simulink model "Battery_Model"  (R2025b)
settings: Solver=VariableStepAuto  StartTime=0.0  StopTime=3000  MaxStep=0.1  MinStep=0.0001  RelTol=1e-3
undefined symbols (not defined in the file or in its folder): DiscIntNeverNeededParam
settings Model: Creator=gonza  LastModifiedBy=gonza

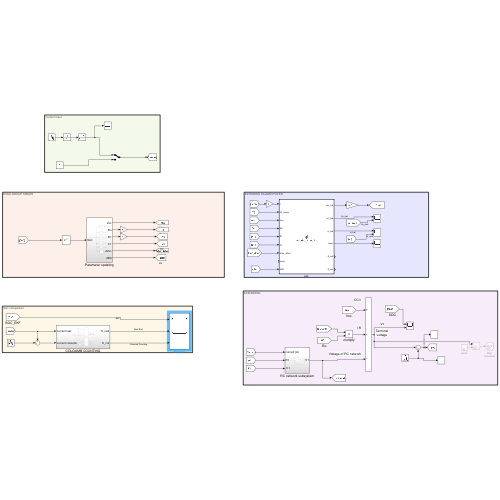
[thumbnail: Simulink's stored preview of the top-level diagram]
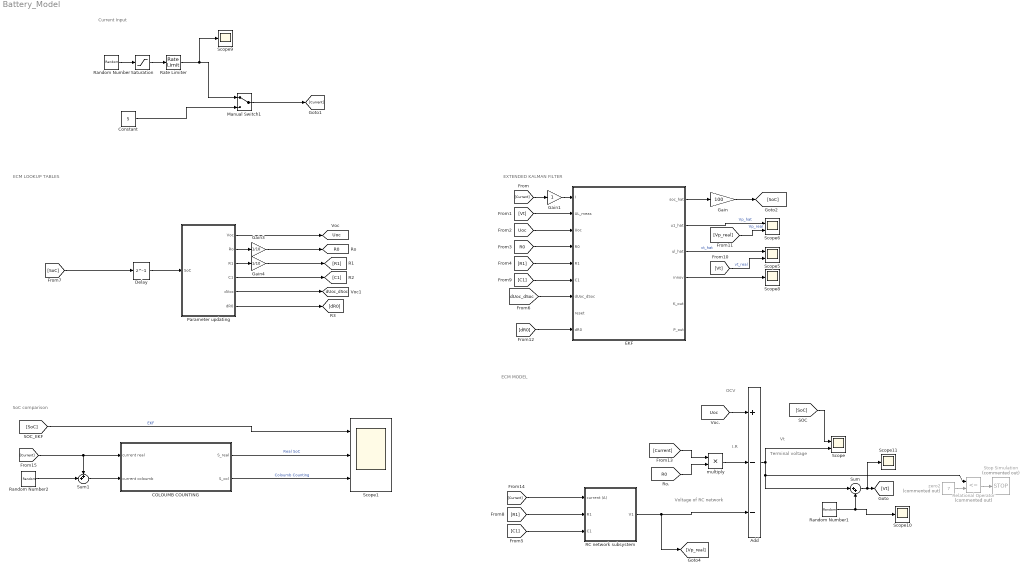
== system Battery_Model ==
  note: SoC comparison
  note: ECM MODEL
  note: Current Input
  note: ECM LOOKUP TABLES
  note: EXTENDED KALMAN FILTER
  note: OCV
  note: Terminal
      |  voltage
  note: Voltage of RC network
  note: Vt
  note: I.R
  Add : Sum  Inputs=+--
  COLOUMB COUNTING : Subsystem
  Constant : Constant  Value=5
  Delay : Delay  DelayLength=1  InitialCondition=80  InputProcessing=Columns as channels (frame based)
  EKF : MATLAB Function  TreatAsAtomicUnit=on
  Gain : Gain  Gain=100
  Gain1 : Gain
  Gain3 : Gain  Gain=1/10
  Gain4 : Gain  Gain=1/10
  Manual Switch1 : ManualSwitch
  Parameter updating : Subsystem
  RC network subsystem : Subsystem
  Random Number : RandomNumber  Variance=100  SampleTime=5
  Random Number1 : RandomNumber  Variance=0.00001  Seed=10  SampleTime=0.01
  Random Number2 : RandomNumber  Variance=0.01  Seed=123412  SampleTime=0.01
  Rate Limiter : RateLimiter  RisingSlewLimit=100  FallingSlewLimit=-100
  Relational Operator : RelationalOperator  Commented=on  Operator=<=  OutDataTypeStr=boolean  InputSameDT=off
  Saturation : Saturate  UpperLimit=100  LowerLimit=-1
  Scope : Scope  NumInputPorts=2
      settings: ActiveDisplayYMinimum=-7.8038423076394752  ActiveDisplayYMaximum=89.71598082300477
  Scope1 : Scope  NumInputPorts=3
      settings: ActiveDisplayYMinimum=5.9960554077224213  ActiveDisplayYMaximum=88.222660510253064
  Scope{8..11} (4 alike) : Scope
      Scope10 settings: ActiveDisplayYMinimum=-0.017996200767772353  ActiveDisplayYMaximum=0.017647380035145821  DataLoggingVariableName=ScopeData10
      Scope11 settings: ActiveDisplayYMinimum=7.0317837281458875  ActiveDisplayYMaximum=7.8836427087263461  DataLoggingVariableName=ScopeData11
      Scope8 settings: ActiveDisplayYMinimum=-0.017332160959111498  ActiveDisplayYMaximum=0.016983840592250665  DataLoggingVariableName=ScopeData8
      Scope9 settings: ActiveDisplayYMinimum=-7.4624542671868479  ActiveDisplayYMaximum=23.142723507063309  DataLoggingVariableName=ScopeData9
  Scope5 : Scope  NumInputPorts=2
      settings: ActiveDisplayYMinimum=7.1842164891272571  ActiveDisplayYMaximum=7.98783766896863  DataLoggingVariableName=ScopeData5
  Scope6 : Scope  NumInputPorts=2
      settings: ActiveDisplayYMinimum=-0.0084839213010874728  ActiveDisplayYMaximum=0.076355291709787276  DataLoggingVariableName=ScopeData6
  Stop Simulation : Stop  Commented=on
  Sum : Sum  Inputs=|++
  Sum1 : Sum  Inputs=++|
  multiply : Product  Inputs=**
  zero2 : Constant  Commented=on  Value=7
  tag scope: R0=global, Uoc=global, dUoc_dSoc=global
  wires:
  EKF/4(innov) -> Scope8/1
  Gain1/1 -> EKF/1(I)
  [dUoc_dSoc] -> EKF/7(dUoc_dSoc)
  EKF/1(soc_hat) -> Gain/1
  Gain/1 -> [SoC]
  [Current] -> Gain1/1
  [R0] -> EKF/4(R0)
  [Vt] -> EKF/2(UL_meas)
  [dR0] -> EKF/9(dR0)
  [C1] -> EKF/6(C1)
  [R1] -> EKF/5(R1)
  EKF/2(u1_hat) -> Scope6/1  "Vp_hat"
  EKF/3(ul_hat) -> Scope5/1  "vt_hat"
  [Vt] -> Scope5/2  "vt_real"
  [Vp_real] -> Scope6/2  "Vp_real"
  [Uoc] -> EKF/3(Uoc)
  Parameter updating/2(Ro) -> Gain3/1
  Gain3/1 -> [R0]
  Parameter updating/1(Voc) -> [Uoc]
  Parameter updating/3(R1) -> Gain4/1
  Gain4/1 -> [R1]
  Parameter updating/5(dVoc) -> [dUoc_dSoc]
  Parameter updating/6(dR0) -> [dR0]
  [SoC] -> Delay/1
  Parameter updating/4(C1) -> [C1]
  Delay/1 -> Parameter updating/1(SoC)
  Constant/1 -> Manual Switch1/2
  Random Number/1 -> Saturation/1
  Saturation/1 -> Rate Limiter/1
  Manual Switch1/1 -> [Current]
  Rate Limiter/1 -> Scope9/1, Manual Switch1/1
  [Current] -> RC network subsystem/1(current (A))
  zero2/1 -> Relational Operator/2
  [R0] -> multiply/2
  [Uoc] -> Add/1
  Random Number1/1 -> Sum/2, Scope10/1
  Add/1 -> Relational Operator/1, Sum/1, Scope/2
  [SoC] -> Scope/1
  multiply/1 -> Add/2
  Sum/1 -> Scope11/1, [Vt]
  Relational Operator/1 -> Stop Simulation/1
  [Current] -> multiply/1
  [R1] -> RC network subsystem/2(R1)
  [C1] -> RC network subsystem/3(" C1")
  RC network subsystem/1(V1) -> Add/3, [Vp_real]
  Sum1/1 -> COLOUMB COUNTING/2(current coloumb)
  Random Number2/1 -> Sum1/2
  [SoC] -> Scope1/1  "EKF"
  [Current] -> Sum1/1, COLOUMB COUNTING/1(current real)
  COLOUMB COUNTING/1(S_real) -> Scope1/2  "Real SoC"
  COLOUMB COUNTING/2(S_col) -> Scope1/3  "Coloumb Counting"

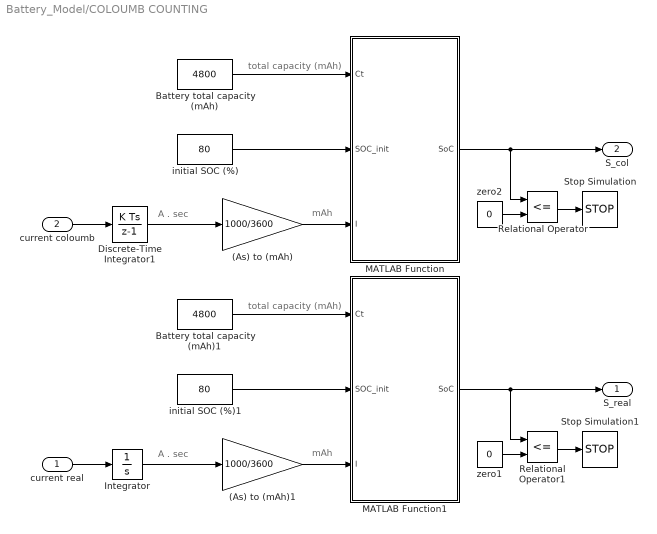
== system Battery_Model/COLOUMB COUNTING ==
  note: total capacity (mAh)
  note: A . sec
  note: mAh
  note: A . sec
  note: total capacity (mAh)
  note: mAh
  current real : Inport
  current coloumb : Inport  Port=2
  (As) to (mAh) : Gain  Gain=1000/3600
  (As) to (mAh)1 : Gain  Gain=1000/3600
  Battery total capacity (mAh) : Constant  Value=4800
  Battery total capacity (mAh)1 : Constant  Value=4800
  Discrete-Time Integrator1 : DiscreteIntegrator  ICPrevOutput=DiscIntNeverNeededParam  ICPrevScaledInput=DiscIntNeverNeededParam
  Integrator : Integrator
  MATLAB Function : MATLAB Function  TreatAsAtomicUnit=on
  MATLAB Function1 : MATLAB Function  TreatAsAtomicUnit=on
  Relational Operator : RelationalOperator  Operator=<=  OutDataTypeStr=boolean  InputSameDT=off
  Relational Operator1 : RelationalOperator  Operator=<=  OutDataTypeStr=boolean  InputSameDT=off
  Stop Simulation : Stop
  Stop Simulation1 : Stop
  initial SOC (%) : Constant  Value=80
  initial SOC (%)1 : Constant  Value=80
  zero1 : Constant  Value=0
  zero2 : Constant  Value=0
  S_real : Outport
  S_col : Outport  Port=2
  wires:
  MATLAB Function/1(SoC) -> S_col/1, Relational Operator/1
  (As) to (mAh)/1 -> MATLAB Function/3(I)
  current coloumb/1 -> Discrete-Time Integrator1/1
  Relational Operator/1 -> Stop Simulation/1
  Battery total capacity (mAh)/1 -> MATLAB Function/1(Ct)
  initial SOC (%)/1 -> MATLAB Function/2(SOC_init)
  zero2/1 -> Relational Operator/2
  zero1/1 -> Relational Operator1/2
  Relational Operator1/1 -> Stop Simulation1/1
  initial SOC (%)1/1 -> MATLAB Function1/2(SOC_init)
  current real/1 -> Integrator/1
  Battery total capacity (mAh)1/1 -> MATLAB Function1/1(Ct)
  (As) to (mAh)1/1 -> MATLAB Function1/3(I)
  MATLAB Function1/1(SoC) -> S_real/1, Relational Operator1/1
  Integrator/1 -> (As) to (mAh)1/1
  Discrete-Time Integrator1/1 -> (As) to (mAh)/1

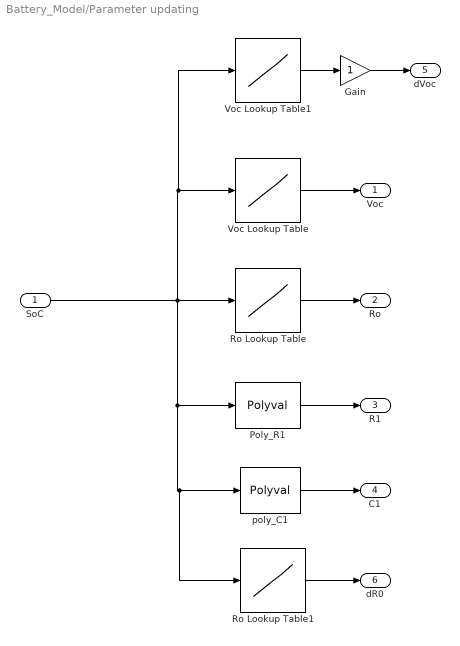
== system Battery_Model/Parameter updating ==
  SoC : Inport
  Gain : Gain
  Poly_R1 : Polyval  Coefs=[1.466124009149211e-08,-3.016114306306107e-06,2.169854530489312e-04,-0.006504304448579,0.091010234125850]
  Ro Lookup Table : Lookup_n-D  NumberOfTableDimensions=1  BreakpointsForDimension1="[0\t5\t7\t9\t11\t13\t15\t17\t19\t21\t23\t25\t27\t29\t31\t33\t35\t37\t39\t41\t43\t45\t47\t49\t51\t53\t55\t57\t59\t61\t63\t65\t67\t69\t71\t73\t75\t77\t79\t81\t83\t85\t87\t89\t91\t93\t95\t97\t100]"  Table="[0.140000000000000\t0.110000000000000\t0.110000000000000\t0.100000000000000\t0.0900000000000000\t0.0900000000000000\t0.0800000000000000\t0.0800000000000000\t0.0700000000000000\t0.0700000000000000\t0.0700000000000000\t0.0700000000000000\t0.0700000000000000\t0.0700000000000000\t0.0700000000000000\t0.0700000000000000\t0.0700000000000000\t0.0600000000000000\t0.0700000000000000\t0.0600000000000000\t0.0600000000000000\t0.0700000000000000\t0.0600000000000000\t0.0700000000000000\t0.0610000000000000\t0.0620000000000000\t0.0630000000000000\t0.0640000000000000\t0.0660000000000000\t0.0650000000000000\t0.0670000000000000\t0.0610000000000000\t0.0610000000000000\t0.0620000000000000\t0.0630000000000000\t0.0620000000000000\t0.0640000000000000\t0.0640000000000000\t0.0650000000000000\t0.0640000000000000\t0.0680000000000000\t0.0710000000000000\t0.0710000000000000\t0.0720000000000000\t0.0740000000000000\t0.0740000000000000\t0.0740000000000000\t0.0750000000000000\t0.0770000000000000]"  InternalRulePriority=Speed  RndMeth=Simplest
  Ro Lookup Table1 : Lookup_n-D  NumberOfTableDimensions=1  BreakpointsForDimension1=[0 5 7 9 11 13 15 17 19 21 23 25 27 29 31 33 35 37 39 41 43 45 47 49 51 53 55 57 59 61 63 65 67 69 71 73 75 77 79 81 83 85 87 89 91 93 95 97 100]  Table=[-0.59999999999999998 -0.42857142857142899 -0.25 -0.5 -0.25 -0.25 -0.25 -0.25 -0.25 0 0 0 0 0 0 0 -0.25 0 0 -0.25 0.25 0 0 0.025000000000000001 -0.20000000000000001 0.050000000000000003 0.050000000000000003 0.074999999999999997 0.025000000000000001 0.025000000000000001 -0.10000000000000001 -0.14999999999999999 0.025000000000000001 0.050000000000000003 0 0.025000000000000001 0.050000000000000003 0.025000000000000001 0 0.074999999999999997 0.17499999999999999 0.074999999999999997 0.025000000000000001 0.074999999999999997 0.050000000000000003 0 0.025000000000000001 0.059999999999999998 0.066666666666666999]  InternalRulePriority=Speed  RndMeth=Simplest
  Voc Lookup Table : Lookup_n-D  NumberOfTableDimensions=1  BreakpointsForDimension1="[0\t5\t7\t9\t11\t13\t15\t17\t19\t21\t23\t25\t27\t29\t31\t33\t35\t37\t39\t41\t43\t45\t47\t49\t51\t53\t55\t57\t59\t61\t63\t65\t67\t69\t71\t73\t75\t77\t79\t81\t83\t85\t87\t89\t91\t93\t95\t97\t100]"  Table="[7.01000000000000\t7.09000000000000\t7.16000000000000\t7.20000000000000\t7.29000000000000\t7.34000000000000\t7.38000000000000\t7.41000000000000\t7.44000000000000\t7.47000000000000\t7.49000000000000\t7.52000000000000\t7.54000000000000\t7.56000000000000\t7.58000000000000\t7.60000000000000\t7.61000000000000\t7.63000000000000\t7.64000000000000\t7.65000000000000\t7.66000000000000\t7.67000000000000\t7.68000000000000\t7.69000000000000\t7.69800000000000\t7.70200000000000\t7.71100000000000\t7.71400000000000\t7.72000000000000\t7.72800000000000\t7.73500000000000\t7.74000000000000\t7.74500000000000\t7.75400000000000\t7.75800000000000\t7.76100000000000\t7.76800000000000\t7.77500000000000\t7.77800000000000\t7.79000000000000\t7.80900000000000\t7.85100000000000\t7.87000000000000\t7.92300000000000\t7.98100000000000\t8.05500000000000\t8.15200000000000\t8.26600000000000\t8.44300000000000]"  InternalRulePriority=Speed  RndMeth=Simplest
  Voc Lookup Table1 : Lookup_n-D  NumberOfTableDimensions=1  BreakpointsForDimension1=[0 5 7 9 11 13 15 17 19 21 23 25 27 29 31 33 35 37 39 41 43 45 47 49 51 53 55 57 59 61 63 65 67 69 71 73 75 77 79 81 83 85 87 89 91 93 95 97 100]  Table=[1.600000000000001 2.142857142857148 2.750000000000008 3.249999999999998 3.499999999999991 2.249999999999997 1.750000000000007 1.500000000000012 1.499999999999991 1.249999999999995 1.249999999999995 1.249999999999995 1.000000000000001 1.000000000000001 1 0.750000000000007 0.750000000000007 0.749999999999983 0.500000000000012 0.500000000000012 0.499999999999989 0.49999999999999 0.500000000000012 0.450000000000017 0.299999999999989 0.324999999999997 0.300000000000012 0.224999999999987 0.349999999999983 0.375000000000014 0.300000000000011 0.249999999999994 0.349999999999984 0.324999999999998 0.175000000000014 0.249999999999994 0.350000000000006 0.249999999999994 0.374999999999992 0.775000000000016 1.525000000000001 1.524999999999997 1.8 2.774999999999991 3.299999999999989 4.274999999999992 5.275000000000017 5.820000000000002 5.899999999999982]  InternalRulePriority=Speed  RndMeth=Simplest
  poly_C1 : Polyval  Coefs=[-6.954272499766545e-05,0.013572818088594,-0.971124742038101,33.500516588178876,92.374565325126170]
  Voc : Outport
  Ro : Outport  Port=2
  R1 : Outport  Port=3
  C1 : Outport  Port=4
  dVoc : Outport  Port=5
  dR0 : Outport  Port=6
  wires:
  SoC/1 -> Ro Lookup Table1/1, poly_C1/1, Poly_R1/1, Voc Lookup Table1/1, Voc Lookup Table/1, Ro Lookup Table/1
  Voc Lookup Table/1 -> Voc/1
  Ro Lookup Table/1 -> Ro/1
  Poly_R1/1 -> R1/1
  poly_C1/1 -> C1/1
  Voc Lookup Table1/1 -> Gain/1
  Gain/1 -> dVoc/1
  Ro Lookup Table1/1 -> dR0/1

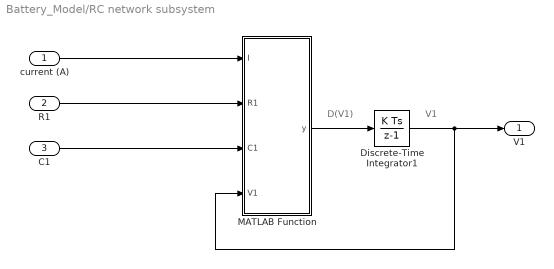
== system Battery_Model/RC network subsystem ==
  note: D(V1)
  note: V1
  current (A) : Inport
  R1 : Inport  Port=2
  " C1" : Inport  Port=3
  Discrete-Time Integrator1 : DiscreteIntegrator  SampleTime=-1  ICPrevOutput=DiscIntNeverNeededParam  ICPrevScaledInput=DiscIntNeverNeededParam
  MATLAB Function : MATLAB Function  TreatAsAtomicUnit=on
  V1 : Outport
  wires:
  MATLAB Function/1(y) -> Discrete-Time Integrator1/1
  Discrete-Time Integrator1/1 -> MATLAB Function/4(V1), V1/1
  current (A)/1 -> MATLAB Function/1(I)
  R1/1 -> MATLAB Function/2(R1)
  " C1"/1 -> MATLAB Function/3(C1)

== matlab function Battery_Model/EKF ==
  settings: updateMethod=DISCRETE
  data: I input; soc_hat output; UL_meas input; Uoc input; R0 input; R1 input; C1 input; dUoc_dSoc input; reset input; u1_hat output; ul_hat output; innov output; K_out output; P_out output; dR0 input
function [soc_hat, u1_hat, ul_hat, innov, K_out, P_out] = soc_ekf_paper_1rc(I, UL_meas, Uoc, R0, R1, C1, dUoc_dSoc, reset,dR0)

    persistent x_hat P initialized


    Dt  = 0.01;         
    Q0  = 3600 * 4.8;   
    
    Qekf = [1e-8, 0;
            0,    1e-8];

    Rekf = 1e-2;


    if isempty(initialized) || reset
        x_hat = [0.8;
                 0.0];

        P = [1e-6, 0;
             0,    1e-6];

        initialized = true;
    end

    SOC_k = x_hat(1);
    U1_k  = x_hat(2);
    SOC_k = min(max(SOC_k, 0.0), 1.0);


    tau1 = R1 * C1;
    a1 = exp(-Dt / tau1);

    A = [1,  0;
         0, a1];

    B = [-Dt / Q0;
         R1 * (1 - exp(-(Dt/tau1)))];

    % =========================================================
    % (1) STATE PREDICTION
    % X(k|k-1) = A X(k-1|k-1) + B U(k-1)
    % =========================================================
    x_pred = A * x_hat + B * I;

    

    
    % (2) COVARIANCE PREDICTION
    % P(k|k-1) = A P(k-1) A' + Q
    
    P_pred = A * P * A.' + Qekf;

    
    % (3) MEASUREMENT JACOBIAN
    % C(k) = dg/dx = [dUoc/dSOC, 1]
    
    C = [dUoc_dSoc-dR0*I, -1];

    
    % PREDICTED OUTPUT
    % UL(k) = Uoc(SOC(k)) + I(k)R0 + U1(k)
    
    ul_hat = Uoc - R0 * I - x_pred(2);

    
    % (4) KALMAN GAIN
    % K = P C' (C P C' + R)^(-1)
   
    S = C * P_pred * C.' + Rekf;
  

    K = (P_pred * C.') / S;

    
    % (5) STATE UPDATE
    % X(k|k) = X(k|k-1) + K [ Z(k) - g(X(k),U(k)) ]
    
    innov = UL_meas - ul_hat;

    x_hat = x_pred + K * innov;
    

    
    % (6) COVARIANCE UPDATE
    % P(k|k) = [I - K C] P(k|k-1)
  
    I2 = eye(2);
    %P = (I2 - K*C) * P_pred * (I2 - K*C).' + K*Rekf*K.';
    P = (I2 - K*C) * P_pred ;

    % Outputs
    soc_hat = x_hat(1);
    u1_hat  = x_hat(2);
    K_out   = K;
    P_out   = P;
end

== matlab function Battery_Model/RC network subsystem/MATLAB Function ==
  data: I input; y output; R1 input; C1 input; V1 input
function y = fcn(I,R1,C1,V1)

y = -V1/(R1*C1)+I/C1;

== matlab function Battery_Model/COLOUMB COUNTING/MATLAB Function ==
  data: Ct input; SoC output; SOC_init input; I input
function SoC = fcn(Ct,SOC_init,I)

% Ct : Battery total capacity (mAh)
% SOC_init : Initial SoC (%)
% I : Cumulative Current (used capacity in mAh)
% y : SoC

 SoC = SOC_init - 100*(I/Ct) ;

end

== matlab function Battery_Model/COLOUMB COUNTING/MATLAB Function1 ==
  data: Ct input; SoC output; SOC_init input; I input
function SoC = fcn(Ct,SOC_init,I)

% Ct : Battery total capacity (mAh)
% SOC_init : Initial SoC (%)
% I : Cumulative Current (used capacity in mAh)
% y : SoC

 SoC = SOC_init - 100*(I/Ct) ;

end
